simulink model "Q2_NORM_MIT"  (R2021b)
settings: Solver=ode45  StartTime=0.0  StopTime=500  FixedStep=.1  RelTol=1e-3  EnableMultiTasking=on
settings Model: Creator=Mehdi  LastModifiedBy=YSNsec
settings SolverCC: AlgebraicLoopSolver=TrustRegion
settings DataIOCC: LimitDataPoints=on  SaveFormat=Array  SignalLoggingSaveFormat=ModelDataLogs  ReturnWorkspaceOutputs=off
settings OptimizationCC: LifeSpan=inf
settings DebuggingCC: UnderspecifiedInitializationDetection=Classic  MergeDetectMultiDrivingBlocksExec=none  MultiTaskDSMMsg=warning  MultiTaskCondExecSysMsg=none  SFUnexpectedBacktrackingDiag=warning  SFNoUnconditionalDefaultTransitionDiag=warning  SFExecutionAtInitializationDiag=none  SFMachineParentedDataDiag=warning  ArithmeticOperatorsInVariantConditions=warning
settings HardwareCC: ProdBitPerPointer=32  ProdBitPerSizeT=32  ProdBitPerPtrDiffT=32  ProdLargestAtomicFloat=None  ProdIntDivRoundTo=Undefined  ProdEndianess=Unspecified  ProdWordSize=32  ProdHWDeviceType=32-bit Generic
settings ModelReferenceCC: PropagateSignalLabelsOutOfModel=off
settings SFSimCC: SimUseLocalCustomCode=off  CustomCodeUndefinedFunction=UseInterfaceOnly
settings RTWCC: RTWUseLocalCustomCode=off
settings CodeAppCC: StateflowObjectComments=on
settings GRTTargetCC: TargetLangStandard=C89/C90 (ANSI)
settings ConfigComp: CovMetricSettings=dw  CovSaveCumulativeToWorkspaceVar=on  CovSaveSingleToWorkspaceVar=on  CovExternalEMLEnable=off

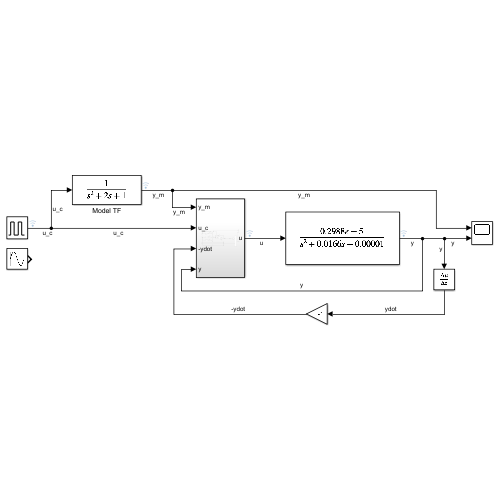
[thumbnail: Simulink's stored preview of the top-level diagram]
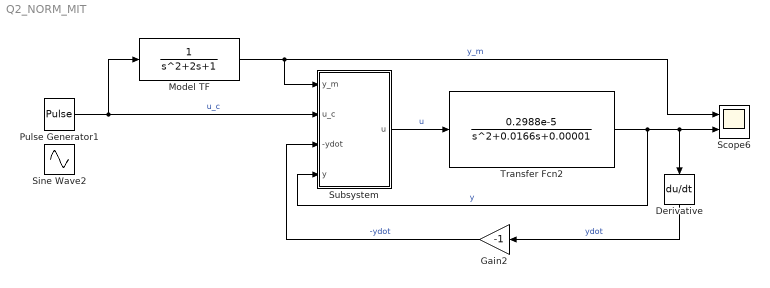
== system Q2_NORM_MIT ==
  Derivative : Derivative
  Gain2 : Gain  Gain=-1
  Model TF : TransferFcn  Numerator=1
  Pulse Generator1 : DiscretePulseGenerator  PulseType=Time based  Amplitude=10  Period=200  PulseWidth=50
  Scope6 : Scope  NumInputPorts=2
  Sine Wave2 : Sin  Amplitude=10  Frequency=0.01  SampleTime=0
  Subsystem : Subsystem
  Transfer Fcn2 : TransferFcn  Numerator=0.2988e-5  Denominator=[1 0.0166 0.00001]
  wires:
  Model TF/1 -> Scope6/1, Subsystem/1(y_m)  "y_m"
  Derivative/1 -> Gain2/1  "ydot"
  Transfer Fcn2/1 -> Scope6/2, Derivative/1, Subsystem/4(y)  "y"
  Pulse Generator1/1 -> Model TF/1, Subsystem/2(u_c)  "u_c"
  Gain2/1 -> Subsystem/3(-ydot)  "-ydot"
  Subsystem/1(u) -> Transfer Fcn2/1  "u"

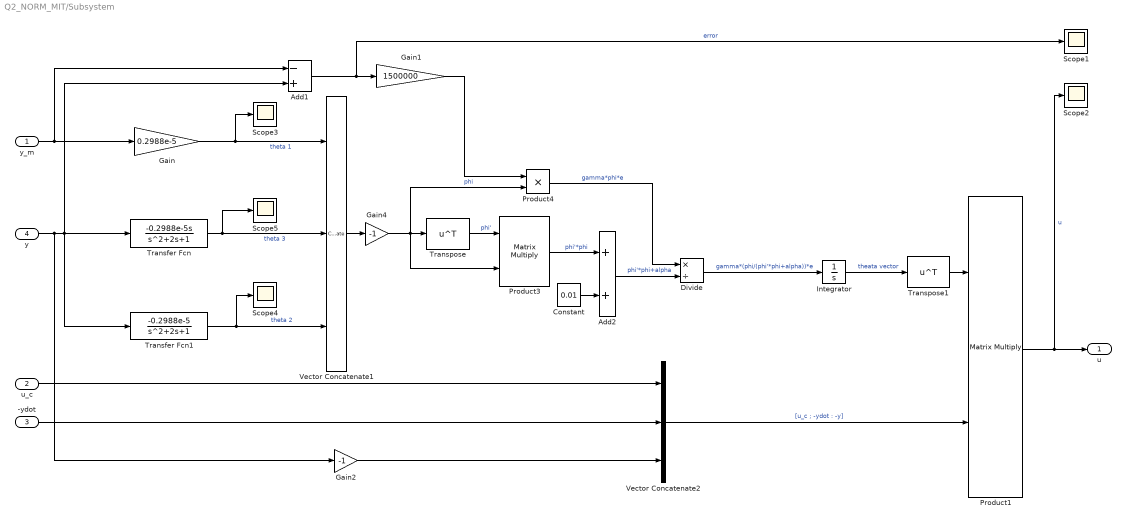
== system Q2_NORM_MIT/Subsystem ==
  y_m : Inport
  u_c : Inport  Port=2
  -ydot : Inport  Port=3
  y : Inport  Port=4
  Add1 : Sum  Inputs=-+
  Add2 : Sum
  Constant : Constant  Value=0.01
  Divide : Product  Inputs=*/
  Gain : Gain  Gain=0.2988e-5
  Gain1 : Gain  Gain=1500000
  Gain2 : Gain  Gain=-1
  Gain4 : Gain  Gain=-1
  Integrator : Integrator
  Product1 : Product  Multiplication=Matrix(*)
  Product3 : Product  Multiplication=Matrix(*)
  Product4 : Product
  Scope{1..5} (5 alike) : Scope
  Transfer Fcn : TransferFcn  Numerator=[-0.2988e-5 0]
  Transfer Fcn1 : TransferFcn  Numerator=[-0.2988e-5]
  Transpose : Math  Operator=transpose  SaturateOnIntegerOverflow=on
  Transpose1 : Math  Operator=transpose  SaturateOnIntegerOverflow=on
  Vector Concatenate1 : Concatenate  NumInputs=3
  Vector Concatenate2 : Concatenate  NumInputs=3
  u : Outport
  wires:
  Gain/1 -> Scope3/1, Vector Concatenate1/1  "theta 1"
  y/1 -> Transfer Fcn1/1, Transfer Fcn/1, Add1/2, Gain2/1
  Add1/1 -> Scope1/1, Gain1/1  "error"
  Product3/1 -> Add2/1  "phi'*phi"
  Constant/1 -> Add2/2
  Gain1/1 -> Product4/1
  Gain4/1 -> Product4/2, Product3/2, Transpose/1  "phi"
  Vector Concatenate1/1 -> Gain4/1
  Divide/1 -> Integrator/1  "gamma*(phi/(phi'*phi+alpha))*e"
  Transpose/1 -> Product3/1  "phi'"
  Add2/1 -> Divide/2  "phi'*phi+alpha"
  Transpose1/1 -> Product1/1
  Product1/1 -> u/1, Scope2/1  "u"
  Transfer Fcn/1 -> Scope5/1, Vector Concatenate1/2  "theta 3"
  Integrator/1 -> Transpose1/1  "theata vector"
  Product4/1 -> Divide/1  "gamma*phi*e"
  Transfer Fcn1/1 -> Scope4/1, Vector Concatenate1/3  "theta 2"
  y_m/1 -> Add1/1, Gain/1
  -ydot/1 -> Vector Concatenate2/2
  Vector Concatenate2/1 -> Product1/2  "[u_c ; -ydot : -y]"
  Gain2/1 -> Vector Concatenate2/3
  u_c/1 -> Vector Concatenate2/1
